simulink model "motor_new_model"  (R2019a)
settings: Solver=ode45  StartTime=0.0  StopTime=0.252  RelTol=1e-3
undefined symbols (not defined in the file or in its folder): B, J, K_e, K_t, L, r, T_l
libraries: simulink x3
settings Model: Creator=Qirat  LastModifiedBy=Asus
settings DataIOCC: ReturnWorkspaceOutputs=off
settings DebuggingCC: PregeneratedLibrarySubsystemCodeDiagnostic=none  ArithmeticOperatorsInVariantConditions=warning
settings SFSimCC: SimUseLocalCustomCode=off
settings RTWCC: RTWUseLocalCustomCode=off

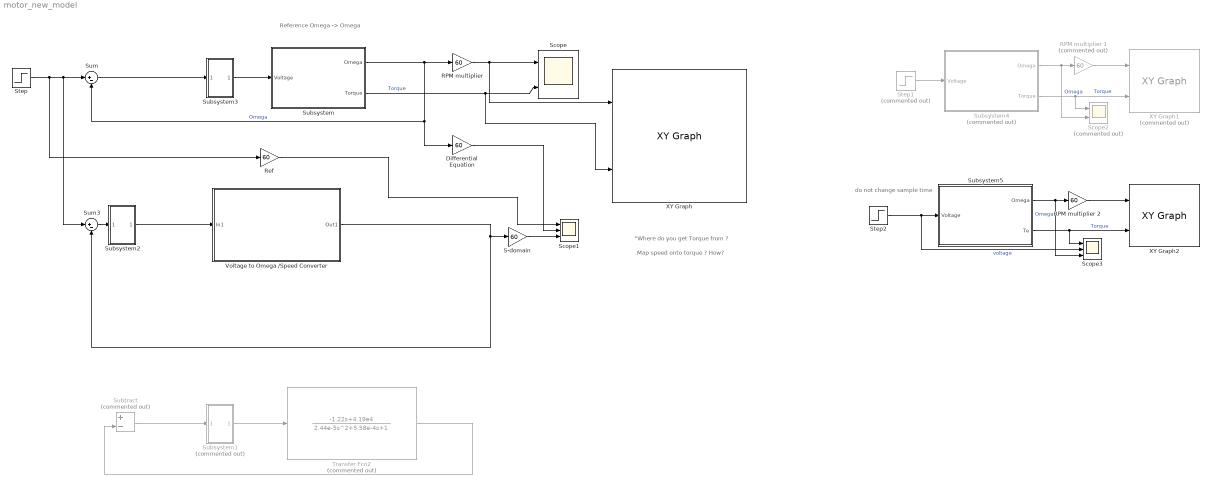
== system motor_new_model ==
  note: do not change sample time
  note: Reference Omega -> Omega
  note: Map speed onto torque ? How?
  note: "Where do you get Torque from ?
  "Differential Equation " : Gain  Gain=60
  "RPM multiplier " : Gain  Gain=60
  RPM multiplier 1 : Gain  Commented=on  Gain=60
  RPM multiplier 2 : Gain  Gain=60
  "Ref " : Gain  Gain=60
  "S-domain " : Gain  Gain=60
  Scope : Scope  NumInputPorts=2
  Scope1 : Scope  NumInputPorts=3
  Scope2 : Scope  Commented=on  NumInputPorts=2
  Scope3 : Scope  NumInputPorts=3
  Step : Step  Time=0.01  After=25  SampleTime=0
  Step1 : Step  Commented=on  After=120  SampleTime=0
  Step2 : Step  Time=0.001  After=30  SampleTime=0
  Subsystem : Subsystem
  Subsystem1 : Subsystem  Commented=on
  Subsystem2 : Subsystem
  Subsystem3 : Subsystem
  Subsystem4 : Subsystem  Commented=on
  Subsystem5 : Subsystem
  Subtract : Sum  Commented=on  Inputs=+-
  Sum : Sum  Inputs=|+-
  Sum3 : Sum  Inputs=|+-
  Transfer Fcn2 : TransferFcn  Commented=on  Numerator=[-1.22 4.19e4]  Denominator=[2.44e-5 5.58e-4 1]
  Voltage to Omega /Speed Converter : Subsystem
  XY Graph : simulink/Sinks/XY Graph  xmin=-1000  xmax=2000  ymin=-1000  ymax=1000  st=0.01
  XY Graph1 : simulink/Sinks/XY Graph  Commented=on  xmin=-1000  xmax=2000  ymin=-1000  ymax=1000  st=0.01
  XY Graph2 : simulink/Sinks/XY Graph  xmin=0  xmax=3500  ymin=0  ymax=2.5  st=0.01
  wires:
  Step/1 -> "Ref "/1, Sum3/1, Sum/1
  Subsystem3/1(Out1) -> Subsystem/1(Voltage)
  Transfer Fcn2/1 -> Subtract/2
  Subtract/1 -> Subsystem1/1(In1)
  Subsystem1/1(Out1) -> Transfer Fcn2/1
  Sum3/1 -> Subsystem2/1(In1)
  Sum/1 -> Subsystem3/1(In1)
  Subsystem/1(Omega) -> "Differential Equation "/1, Sum/2, "RPM multiplier "/1  "Omega"
  "Ref "/1 -> Scope1/1
  "Differential Equation "/1 -> Scope1/2
  "S-domain "/1 -> Scope1/3
  Voltage to Omega /Speed Converter/1(Out1) -> Sum3/2, "S-domain "/1
  Subsystem2/1(Out1) -> Voltage to Omega /Speed Converter/1(In1)
  Subsystem/2("Torque ") -> XY Graph/2, Scope/2  "Torque"
  "RPM multiplier "/1 -> XY Graph/1, Scope/1
  Step1/1 -> Subsystem4/1(Voltage)
  Subsystem4/1(Omega) -> Scope2/2, RPM multiplier 1/1  "Omega"
  RPM multiplier 1/1 -> XY Graph1/1
  Subsystem4/2("Torque ") -> Scope2/1, XY Graph1/2  "Torque"
  Subsystem5/2(Te) -> Scope3/1, XY Graph2/2  "Torque"
  Subsystem5/1(Omega) -> Scope3/3, RPM multiplier 2/1  "Omega"
  RPM multiplier 2/1 -> XY Graph2/1
  Step2/1 -> Scope3/2, Subsystem5/1(Voltage)  "voltage"

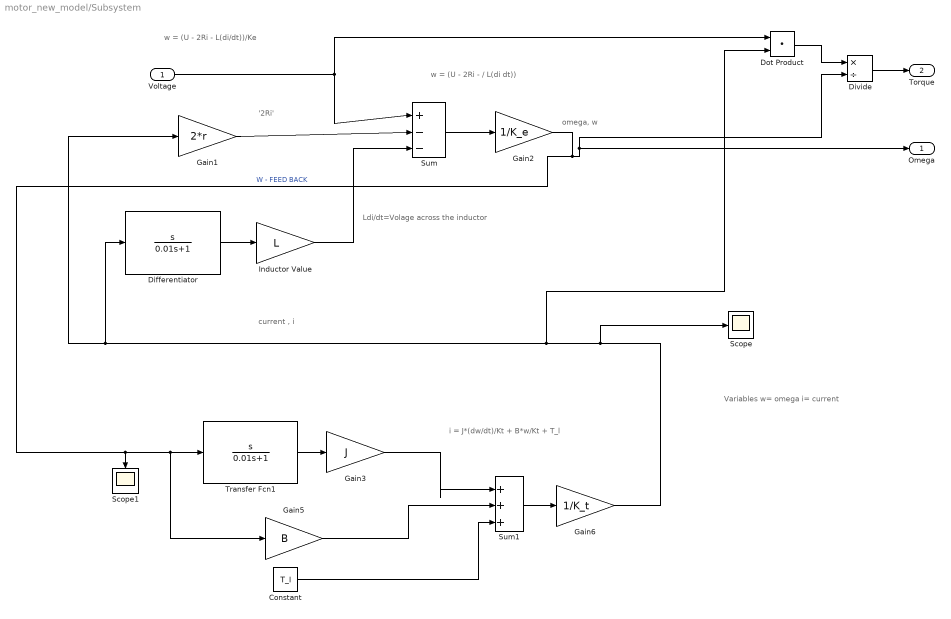
== system motor_new_model/Subsystem ==
  note: Variables
      | w= omega
      | i= current
  note: '2Ri'
  note: current , i
  note: i = J*(dw/dt)/Kt + B*w/Kt + T_l
  note: w = (U - 2Ri - L(di/dt))/Ke
  note: omega, w
  note: w = (U - 2Ri - / L(di dt))
  note: Ldi/dt=Volage across the inductor
  Voltage : Inport
  Constant : Constant  Value=T_l
  "Differentiator " : TransferFcn  Numerator=[1 0]  Denominator=[0.01 1]
  Divide : Product  Inputs=*/
  Dot Product : DotProduct  InputSameDT=on  OutDataTypeStr=Inherit: Inherit via internal rule
  Gain1 : Gain  Gain=2*r
  Gain2 : Gain  Gain=1/K_e
  Gain3 : Gain  Gain=J
  Gain5 : Gain  Gain=B
  Gain6 : Gain  Gain=1/K_t
  Inductor Value : Gain  Gain=L
  Scope : Scope
  Scope1 : Scope
  Sum : Sum  Inputs=|+--
  Sum1 : Sum  Inputs=|+++
  Transfer Fcn1 : TransferFcn  Numerator=[1 0]  Denominator=[0.01 1]
  Omega : Outport
  "Torque " : Outport  Port=2
  wires:
  Gain1/1 -> Sum/2
  Sum/1 -> Gain2/1
  Gain2/1 -> Scope1/1, Transfer Fcn1/1, Gain5/1, Divide/2, Omega/1  "W - FEED BACK"
  Voltage/1 -> Dot Product/1, Sum/1
  Transfer Fcn1/1 -> Gain3/1
  "Differentiator "/1 -> Inductor Value/1
  Inductor Value/1 -> Sum/3
  Gain3/1 -> Sum1/1
  Gain5/1 -> Sum1/2
  Sum1/1 -> Gain6/1
  Gain6/1 -> Dot Product/2, Gain1/1, "Differentiator "/1, Scope/1
  Constant/1 -> Sum1/3
  Dot Product/1 -> Divide/1
  Divide/1 -> "Torque "/1

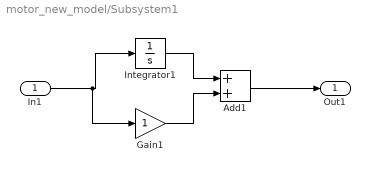
== system motor_new_model/Subsystem1 ==
  In1 : Inport
  Add1 : Sum
  Gain1 : Gain
  Integrator1 : Integrator
  Out1 : Outport
  wires:
  Integrator1/1 -> Add1/1
  In1/1 -> Gain1/1, Integrator1/1
  Gain1/1 -> Add1/2
  Add1/1 -> Out1/1

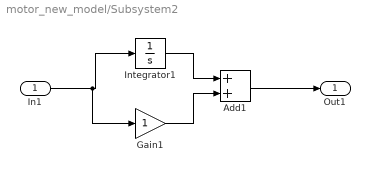
== system motor_new_model/Subsystem2 ==
  In1 : Inport
  Add1 : Sum
  Gain1 : Gain
  Integrator1 : Integrator
  Out1 : Outport
  wires:
  Integrator1/1 -> Add1/1
  In1/1 -> Gain1/1, Integrator1/1
  Gain1/1 -> Add1/2
  Add1/1 -> Out1/1

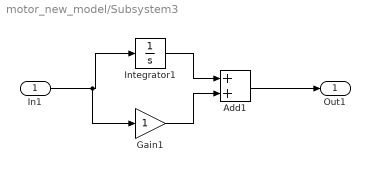
== system motor_new_model/Subsystem3 ==
  In1 : Inport
  Add1 : Sum
  Gain1 : Gain
  Integrator1 : Integrator
  Out1 : Outport
  wires:
  Integrator1/1 -> Add1/1
  In1/1 -> Gain1/1, Integrator1/1
  Gain1/1 -> Add1/2
  Add1/1 -> Out1/1

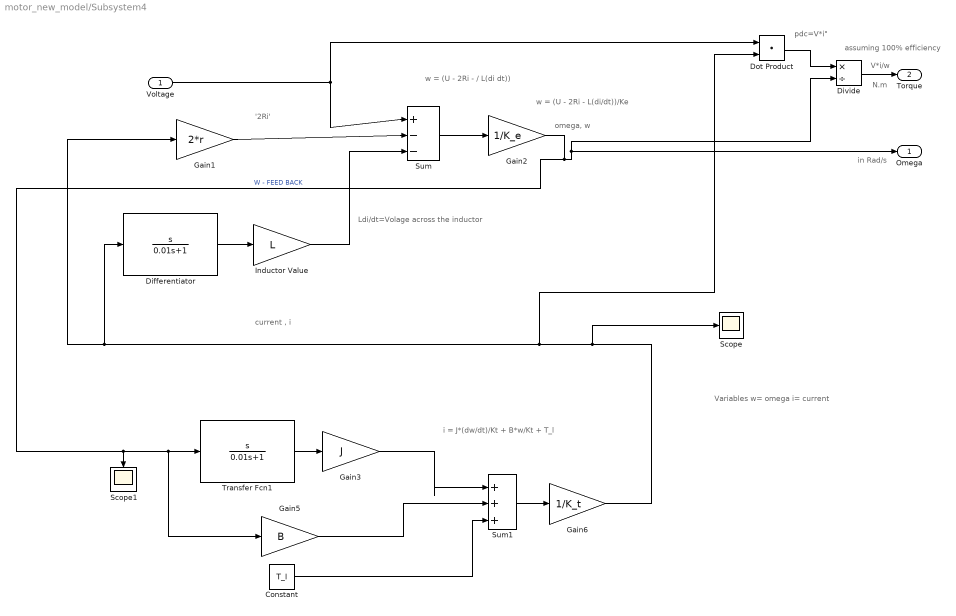
== system motor_new_model/Subsystem4 ==
  note: assuming 100% efficiency
  note: N.m
  note: in Rad/s
  note: pdc=V*i"
  note: Variables
      | w= omega
      | i= current
  note: '2Ri'
  note: current , i
  note: i = J*(dw/dt)/Kt + B*w/Kt + T_l
  note: w = (U - 2Ri - L(di/dt))/Ke
  note: omega, w
  note: w = (U - 2Ri - / L(di dt))
  note: Ldi/dt=Volage across the inductor
  note: V*i/w
  Voltage : Inport
  Constant : Constant  Value=T_l
  "Differentiator " : TransferFcn  Numerator=[1 0]  Denominator=[0.01 1]
  Divide : Product  Inputs=*/
  Dot Product : DotProduct  InputSameDT=on  OutDataTypeStr=Inherit: Inherit via internal rule
  Gain1 : Gain  Gain=2*r
  Gain2 : Gain  Gain=1/K_e
  Gain3 : Gain  Gain=J
  Gain5 : Gain  Gain=B
  Gain6 : Gain  Gain=1/K_t
  Inductor Value : Gain  Gain=L
  Scope : Scope
  Scope1 : Scope
  Sum : Sum  Inputs=|+--
  Sum1 : Sum  Inputs=|+++
  Transfer Fcn1 : TransferFcn  Numerator=[1 0]  Denominator=[0.01 1]
  Omega : Outport
  "Torque " : Outport  Port=2
  wires:
  Gain1/1 -> Sum/2
  Sum/1 -> Gain2/1
  Gain2/1 -> Scope1/1, Transfer Fcn1/1, Gain5/1, Divide/2, Omega/1  "W - FEED BACK"
  Voltage/1 -> Dot Product/1, Sum/1
  Transfer Fcn1/1 -> Gain3/1
  "Differentiator "/1 -> Inductor Value/1
  Inductor Value/1 -> Sum/3
  Gain3/1 -> Sum1/1
  Gain5/1 -> Sum1/2
  Sum1/1 -> Gain6/1
  Gain6/1 -> Dot Product/2, Gain1/1, "Differentiator "/1, Scope/1
  Constant/1 -> Sum1/3
  Dot Product/1 -> Divide/1
  Divide/1 -> "Torque "/1

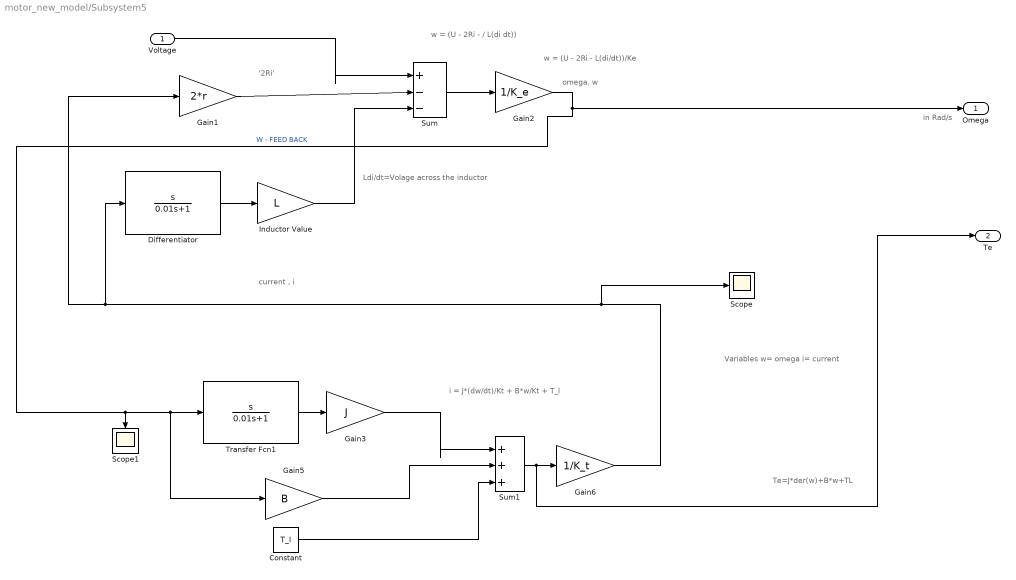
== system motor_new_model/Subsystem5 ==
  note: Te=J*der(w)+B*w+TL
  note: in Rad/s
  note: Variables
      | w= omega
      | i= current
  note: '2Ri'
  note: current , i
  note: i = J*(dw/dt)/Kt + B*w/Kt + T_l
  note: w = (U - 2Ri - L(di/dt))/Ke
  note: omega, w
  note: w = (U - 2Ri - / L(di dt))
  note: Ldi/dt=Volage across the inductor
  Voltage : Inport
  Constant : Constant  Value=T_l
  "Differentiator " : TransferFcn  Numerator=[1 0]  Denominator=[0.01 1]
  Gain1 : Gain  Gain=2*r
  Gain2 : Gain  Gain=1/K_e
  Gain3 : Gain  Gain=J
  Gain5 : Gain  Gain=B
  Gain6 : Gain  Gain=1/K_t
  Inductor Value : Gain  Gain=L
  Scope : Scope
  Scope1 : Scope
  Sum : Sum  Inputs=|+--
  Sum1 : Sum  Inputs=|+++
  Transfer Fcn1 : TransferFcn  Numerator=[1 0]  Denominator=[0.01 1]
  Omega : Outport
  Te : Outport  Port=2
  wires:
  Gain1/1 -> Sum/2
  Sum/1 -> Gain2/1
  Gain2/1 -> Scope1/1, Transfer Fcn1/1, Gain5/1, Omega/1  "W - FEED BACK"
  Voltage/1 -> Sum/1
  Transfer Fcn1/1 -> Gain3/1
  "Differentiator "/1 -> Inductor Value/1
  Inductor Value/1 -> Sum/3
  Gain3/1 -> Sum1/1
  Gain5/1 -> Sum1/2
  Gain6/1 -> Gain1/1, "Differentiator "/1, Scope/1
  Constant/1 -> Sum1/3
  Sum1/1 -> Te/1, Gain6/1

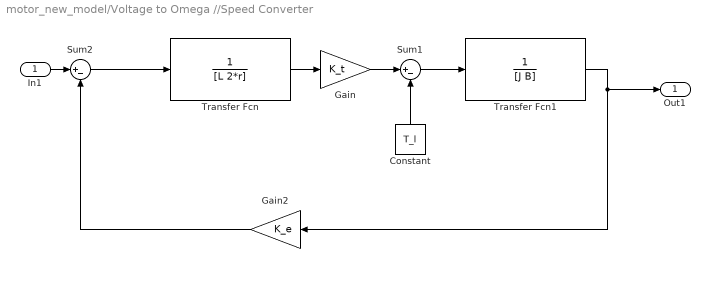
== system motor_new_model/Voltage to Omega //Speed Converter ==
  In1 : Inport
  Constant : Constant  Value=T_l
  Gain : Gain  Gain=K_t
  Gain2 : Gain  Gain=K_e
  Sum1 : Sum  Inputs=|+-
  Sum2 : Sum  Inputs=|+-
  Transfer Fcn : TransferFcn  Denominator=[L 2*r]
  Transfer Fcn1 : TransferFcn  Denominator=[J B]
  Out1 : Outport
  wires:
  Transfer Fcn1/1 -> Out1/1, Gain2/1
  In1/1 -> Sum2/1
  Sum1/1 -> Transfer Fcn1/1
  Gain2/1 -> Sum2/2
  Transfer Fcn/1 -> Gain/1
  Constant/1 -> Sum1/2
  Sum2/1 -> Transfer Fcn/1
  Gain/1 -> Sum1/1
